simulink library "halin"  (R2021b)
settings: Solver=VariableStepAuto  StartTime=0.0  StopTime=10.0  RelTol=1e-3
undefined symbols (not defined in the file): TRUE
libraries: FVT_lib x37, hcu_lib x31
(part 3 of 4)

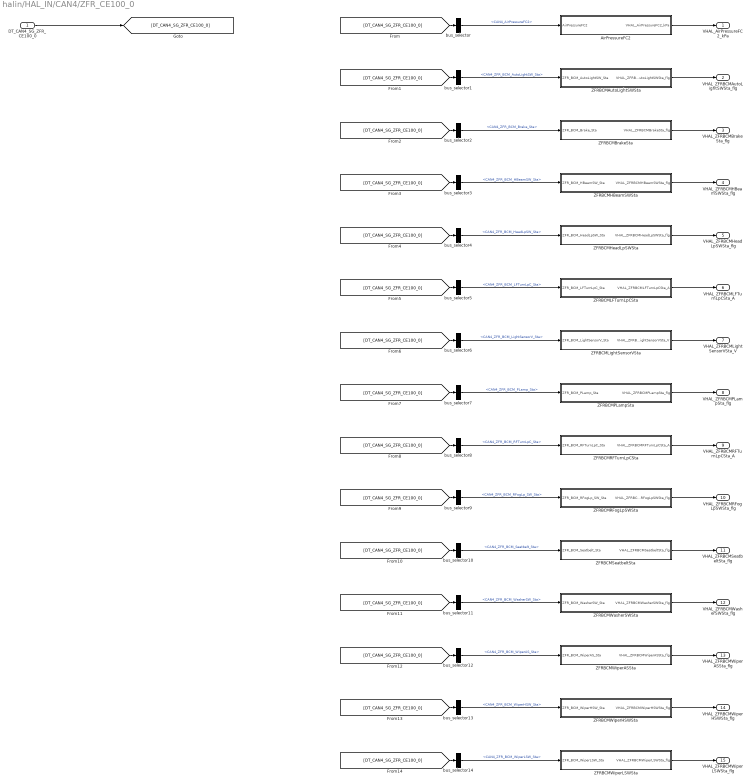
== system halin/HAL_IN/CAN4/ZFR_CE100_0 ==
  DT_CAN4_SG_ZFR_CE100_0 : Inport
  AirPressureFC2 : Subsystem
  ZFRBCMAutoLightSWSta : Subsystem
  ZFRBCMBrakeSta : Subsystem
  ZFRBCMHBeamSWSta : Subsystem
  ZFRBCMHeadLpSWSta : Subsystem
  ZFRBCMLFTurnLpCSta : Subsystem
  ZFRBCMLightSensorVSta : Subsystem
  ZFRBCMPLampSta : Subsystem
  ZFRBCMRFTurnLpCSta : Subsystem
  ZFRBCMRFogLpSWSta : Subsystem
  ZFRBCMSeatbeltSta : Subsystem
  ZFRBCMWasherSWSta : Subsystem
  ZFRBCMWiperASSta : Subsystem
  ZFRBCMWiperHSWSta : Subsystem
  ZFRBCMWiperLSWSta : Subsystem
  bus_selector : BusSelector  OutputSignals=CAN4_AirPressureFC2
  bus_selector1 : BusSelector  OutputSignals=CAN4_ZFR_BCM_AutoLightSW_Sta
  bus_selector10 : BusSelector  OutputSignals=CAN4_ZFR_BCM_Seatbelt_Sta
  bus_selector11 : BusSelector  OutputSignals=CAN4_ZFR_BCM_WasherSW_Sta
  bus_selector12 : BusSelector  OutputSignals=CAN4_ZFR_BCM_WiperAS_Sta
  bus_selector13 : BusSelector  OutputSignals=CAN4_ZFR_BCM_WiperHSW_Sta
  bus_selector14 : BusSelector  OutputSignals=CAN4_ZFR_BCM_WiperLSW_Sta
  bus_selector2 : BusSelector  OutputSignals=CAN4_ZFR_BCM_Brake_Sta
  bus_selector3 : BusSelector  OutputSignals=CAN4_ZFR_BCM_HBeamSW_Sta
  bus_selector4 : BusSelector  OutputSignals=CAN4_ZFR_BCM_HeadLpSW_Sta
  bus_selector5 : BusSelector  OutputSignals=CAN4_ZFR_BCM_LFTurnLpC_Sta
  bus_selector6 : BusSelector  OutputSignals=CAN4_ZFR_BCM_LightSensorV_Sta
  bus_selector7 : BusSelector  OutputSignals=CAN4_ZFR_BCM_PLamp_Sta
  bus_selector8 : BusSelector  OutputSignals=CAN4_ZFR_BCM_RFTurnLpC_Sta
  bus_selector9 : BusSelector  OutputSignals=CAN4_ZFR_BCM_RFogLp_SW_Sta
  VHAL_AirPressureFC2_kPa : Outport
  VHAL_ZFRBCMAutoLightSWSta_flg : Outport  Port=2
  VHAL_ZFRBCMBrakeSta_flg : Outport  Port=3
  VHAL_ZFRBCMHBeamSWSta_flg : Outport  Port=4
  VHAL_ZFRBCMHeadLpSWSta_flg : Outport  Port=5
  VHAL_ZFRBCMLFTurnLpCSta_A : Outport  Port=6
  VHAL_ZFRBCMLightSensorVSta_V : Outport  Port=7
  VHAL_ZFRBCMPLampSta_flg : Outport  Port=8
  VHAL_ZFRBCMRFTurnLpCSta_A : Outport  Port=9
  VHAL_ZFRBCMRFogLpSWSta_flg : Outport  Port=10
  VHAL_ZFRBCMSeatbeltSta_flg : Outport  Port=11
  VHAL_ZFRBCMWasherSWSta_flg : Outport  Port=12
  VHAL_ZFRBCMWiperASSta_flg : Outport  Port=13
  VHAL_ZFRBCMWiperHSWSta_flg : Outport  Port=14
  VHAL_ZFRBCMWiperLSWSta_flg : Outport  Port=15
  wires:
  DT_CAN4_SG_ZFR_CE100_0/1 -> [DT_CAN4_SG_ZFR_CE100_0]
  [DT_CAN4_SG_ZFR_CE100_0] -> bus_selector/1
  bus_selector/1 -> AirPressureFC2/1(AirPressureFC2)  "<CAN4_AirPressureFC2>"
  AirPressureFC2/1(VHAL_AirPressureFC2_kPa) -> VHAL_AirPressureFC2_kPa/1
  [DT_CAN4_SG_ZFR_CE100_0] -> bus_selector1/1
  bus_selector1/1 -> ZFRBCMAutoLightSWSta/1(ZFR_BCM_AutoLightSW_Sta)  "<CAN4_ZFR_BCM_AutoLightSW_Sta>"
  ZFRBCMAutoLightSWSta/1(VHAL_ZFRBCMAutoLightSWSta_flg) -> VHAL_ZFRBCMAutoLightSWSta_flg/1
  [DT_CAN4_SG_ZFR_CE100_0] -> bus_selector2/1
  bus_selector2/1 -> ZFRBCMBrakeSta/1(ZFR_BCM_Brake_Sta)  "<CAN4_ZFR_BCM_Brake_Sta>"
  ZFRBCMBrakeSta/1(VHAL_ZFRBCMBrakeSta_flg) -> VHAL_ZFRBCMBrakeSta_flg/1
  [DT_CAN4_SG_ZFR_CE100_0] -> bus_selector3/1
  bus_selector3/1 -> ZFRBCMHBeamSWSta/1(ZFR_BCM_HBeamSW_Sta)  "<CAN4_ZFR_BCM_HBeamSW_Sta>"
  ZFRBCMHBeamSWSta/1(VHAL_ZFRBCMHBeamSWSta_flg) -> VHAL_ZFRBCMHBeamSWSta_flg/1
  [DT_CAN4_SG_ZFR_CE100_0] -> bus_selector4/1
  bus_selector4/1 -> ZFRBCMHeadLpSWSta/1(ZFR_BCM_HeadLpSW_Sta)  "<CAN4_ZFR_BCM_HeadLpSW_Sta>"
  ZFRBCMHeadLpSWSta/1(VHAL_ZFRBCMHeadLpSWSta_flg) -> VHAL_ZFRBCMHeadLpSWSta_flg/1
  [DT_CAN4_SG_ZFR_CE100_0] -> bus_selector5/1
  bus_selector5/1 -> ZFRBCMLFTurnLpCSta/1(ZFR_BCM_LFTurnLpC_Sta)  "<CAN4_ZFR_BCM_LFTurnLpC_Sta>"
  ZFRBCMLFTurnLpCSta/1(VHAL_ZFRBCMLFTurnLpCSta_A) -> VHAL_ZFRBCMLFTurnLpCSta_A/1
  [DT_CAN4_SG_ZFR_CE100_0] -> bus_selector6/1
  bus_selector6/1 -> ZFRBCMLightSensorVSta/1(ZFR_BCM_LightSensorV_Sta)  "<CAN4_ZFR_BCM_LightSensorV_Sta>"
  ZFRBCMLightSensorVSta/1(VHAL_ZFRBCMLightSensorVSta_V) -> VHAL_ZFRBCMLightSensorVSta_V/1
  [DT_CAN4_SG_ZFR_CE100_0] -> bus_selector7/1
  bus_selector7/1 -> ZFRBCMPLampSta/1(ZFR_BCM_PLamp_Sta)  "<CAN4_ZFR_BCM_PLamp_Sta>"
  ZFRBCMPLampSta/1(VHAL_ZFRBCMPLampSta_flg) -> VHAL_ZFRBCMPLampSta_flg/1
  [DT_CAN4_SG_ZFR_CE100_0] -> bus_selector8/1
  bus_selector8/1 -> ZFRBCMRFTurnLpCSta/1(ZFR_BCM_RFTurnLpC_Sta)  "<CAN4_ZFR_BCM_RFTurnLpC_Sta>"
  ZFRBCMRFTurnLpCSta/1(VHAL_ZFRBCMRFTurnLpCSta_A) -> VHAL_ZFRBCMRFTurnLpCSta_A/1
  [DT_CAN4_SG_ZFR_CE100_0] -> bus_selector9/1
  bus_selector9/1 -> ZFRBCMRFogLpSWSta/1(ZFR_BCM_RFogLp_SW_Sta)  "<CAN4_ZFR_BCM_RFogLp_SW_Sta>"
  ZFRBCMRFogLpSWSta/1(VHAL_ZFRBCMRFogLpSWSta_flg) -> VHAL_ZFRBCMRFogLpSWSta_flg/1
  [DT_CAN4_SG_ZFR_CE100_0] -> bus_selector10/1
  bus_selector10/1 -> ZFRBCMSeatbeltSta/1(ZFR_BCM_Seatbelt_Sta)  "<CAN4_ZFR_BCM_Seatbelt_Sta>"
  ZFRBCMSeatbeltSta/1(VHAL_ZFRBCMSeatbeltSta_flg) -> VHAL_ZFRBCMSeatbeltSta_flg/1
  [DT_CAN4_SG_ZFR_CE100_0] -> bus_selector11/1
  bus_selector11/1 -> ZFRBCMWasherSWSta/1(ZFR_BCM_WasherSW_Sta)  "<CAN4_ZFR_BCM_WasherSW_Sta>"
  ZFRBCMWasherSWSta/1(VHAL_ZFRBCMWasherSWSta_flg) -> VHAL_ZFRBCMWasherSWSta_flg/1
  [DT_CAN4_SG_ZFR_CE100_0] -> bus_selector12/1
  bus_selector12/1 -> ZFRBCMWiperASSta/1(ZFR_BCM_WiperAS_Sta)  "<CAN4_ZFR_BCM_WiperAS_Sta>"
  ZFRBCMWiperASSta/1(VHAL_ZFRBCMWiperASSta_flg) -> VHAL_ZFRBCMWiperASSta_flg/1
  [DT_CAN4_SG_ZFR_CE100_0] -> bus_selector13/1
  bus_selector13/1 -> ZFRBCMWiperHSWSta/1(ZFR_BCM_WiperHSW_Sta)  "<CAN4_ZFR_BCM_WiperHSW_Sta>"
  ZFRBCMWiperHSWSta/1(VHAL_ZFRBCMWiperHSWSta_flg) -> VHAL_ZFRBCMWiperHSWSta_flg/1
  [DT_CAN4_SG_ZFR_CE100_0] -> bus_selector14/1
  bus_selector14/1 -> ZFRBCMWiperLSWSta/1(ZFR_BCM_WiperLSW_Sta)  "<CAN4_ZFR_BCM_WiperLSW_Sta>"
  ZFRBCMWiperLSWSta/1(VHAL_ZFRBCMWiperLSWSta_flg) -> VHAL_ZFRBCMWiperLSWSta_flg/1

== system halin/HAL_IN/CAN4/ZRR_CE100_0 ==
  DT_CAN4_SG_ZRR_CE100_0 : Inport
  ZRRBCMAllDoorSta : Subsystem
  bus_selector : BusSelector  OutputSignals=CAN4_ZRR_BCM_AllDoor_Sta
  VHAL_ZRRBCMAllDoorSta_enum : Outport
  wires:
  DT_CAN4_SG_ZRR_CE100_0/1 -> [DT_CAN4_SG_ZRR_CE100_0]
  [DT_CAN4_SG_ZRR_CE100_0] -> bus_selector/1
  bus_selector/1 -> ZRRBCMAllDoorSta/1(ZRR_BCM_AllDoor_Sta)  "<CAN4_ZRR_BCM_AllDoor_Sta>"
  ZRRBCMAllDoorSta/1(VHAL_ZRRBCMAllDoorSta_enum) -> VHAL_ZRRBCMAllDoorSta_enum/1

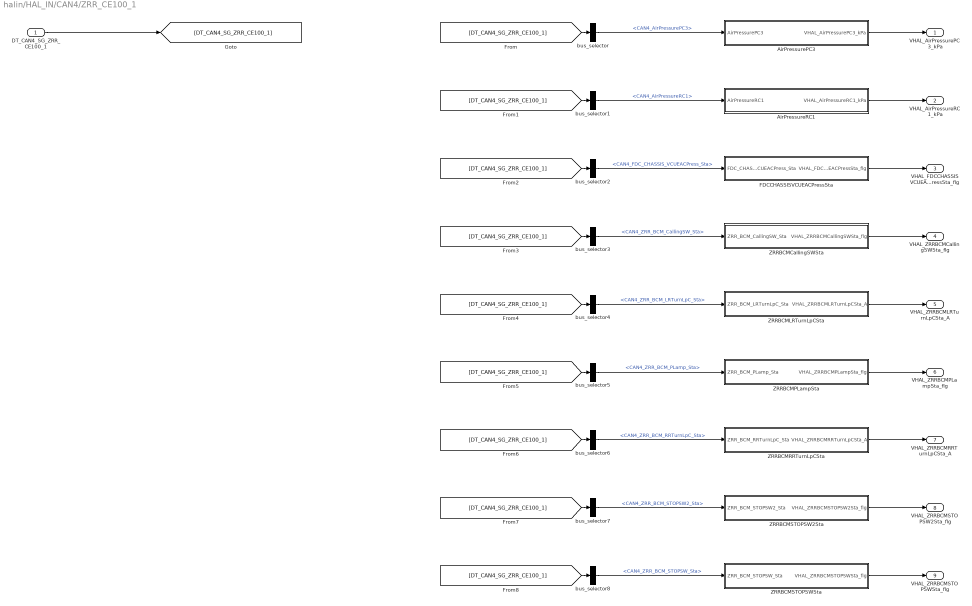
== system halin/HAL_IN/CAN4/ZRR_CE100_1 ==
  DT_CAN4_SG_ZRR_CE100_1 : Inport
  AirPressurePC3 : Subsystem
  AirPressureRC1 : Subsystem
  FDCCHASSISVCUEACPressSta : Subsystem
  ZRRBCMCallingSWSta : Subsystem
  ZRRBCMLRTurnLpCSta : Subsystem
  ZRRBCMPLampSta : Subsystem
  ZRRBCMRRTurnLpCSta : Subsystem
  ZRRBCMSTOPSW2Sta : Subsystem
  ZRRBCMSTOPSWSta : Subsystem
  bus_selector : BusSelector  OutputSignals=CAN4_AirPressurePC3
  bus_selector1 : BusSelector  OutputSignals=CAN4_AirPressureRC1
  bus_selector2 : BusSelector  OutputSignals=CAN4_FDC_CHASSIS_VCUEACPress_Sta
  bus_selector3 : BusSelector  OutputSignals=CAN4_ZRR_BCM_CallingSW_Sta
  bus_selector4 : BusSelector  OutputSignals=CAN4_ZRR_BCM_LRTurnLpC_Sta
  bus_selector5 : BusSelector  OutputSignals=CAN4_ZRR_BCM_PLamp_Sta
  bus_selector6 : BusSelector  OutputSignals=CAN4_ZRR_BCM_RRTurnLpC_Sta
  bus_selector7 : BusSelector  OutputSignals=CAN4_ZRR_BCM_STOPSW2_Sta
  bus_selector8 : BusSelector  OutputSignals=CAN4_ZRR_BCM_STOPSW_Sta
  VHAL_AirPressurePC3_kPa : Outport
  VHAL_AirPressureRC1_kPa : Outport  Port=2
  VHAL_FDCCHASSISVCUEACPressSta_flg : Outport  Port=3
  VHAL_ZRRBCMCallingSWSta_flg : Outport  Port=4
  VHAL_ZRRBCMLRTurnLpCSta_A : Outport  Port=5
  VHAL_ZRRBCMPLampSta_flg : Outport  Port=6
  VHAL_ZRRBCMRRTurnLpCSta_A : Outport  Port=7
  VHAL_ZRRBCMSTOPSW2Sta_flg : Outport  Port=8
  VHAL_ZRRBCMSTOPSWSta_flg : Outport  Port=9
  wires:
  DT_CAN4_SG_ZRR_CE100_1/1 -> [DT_CAN4_SG_ZRR_CE100_1]
  [DT_CAN4_SG_ZRR_CE100_1] -> bus_selector/1
  bus_selector/1 -> AirPressurePC3/1(AirPressurePC3)  "<CAN4_AirPressurePC3>"
  AirPressurePC3/1(VHAL_AirPressurePC3_kPa) -> VHAL_AirPressurePC3_kPa/1
  [DT_CAN4_SG_ZRR_CE100_1] -> bus_selector1/1
  bus_selector1/1 -> AirPressureRC1/1(AirPressureRC1)  "<CAN4_AirPressureRC1>"
  AirPressureRC1/1(VHAL_AirPressureRC1_kPa) -> VHAL_AirPressureRC1_kPa/1
  [DT_CAN4_SG_ZRR_CE100_1] -> bus_selector2/1
  bus_selector2/1 -> FDCCHASSISVCUEACPressSta/1(FDC_CHASSIS_VCUEACPress_Sta)  "<CAN4_FDC_CHASSIS_VCUEACPress_Sta>"
  FDCCHASSISVCUEACPressSta/1(VHAL_FDCCHASSISVCUEACPressSta_flg) -> VHAL_FDCCHASSISVCUEACPressSta_flg/1
  [DT_CAN4_SG_ZRR_CE100_1] -> bus_selector3/1
  bus_selector3/1 -> ZRRBCMCallingSWSta/1(ZRR_BCM_CallingSW_Sta)  "<CAN4_ZRR_BCM_CallingSW_Sta>"
  ZRRBCMCallingSWSta/1(VHAL_ZRRBCMCallingSWSta_flg) -> VHAL_ZRRBCMCallingSWSta_flg/1
  [DT_CAN4_SG_ZRR_CE100_1] -> bus_selector4/1
  bus_selector4/1 -> ZRRBCMLRTurnLpCSta/1(ZRR_BCM_LRTurnLpC_Sta)  "<CAN4_ZRR_BCM_LRTurnLpC_Sta>"
  ZRRBCMLRTurnLpCSta/1(VHAL_ZRRBCMLRTurnLpCSta_A) -> VHAL_ZRRBCMLRTurnLpCSta_A/1
  [DT_CAN4_SG_ZRR_CE100_1] -> bus_selector5/1
  bus_selector5/1 -> ZRRBCMPLampSta/1(ZRR_BCM_PLamp_Sta)  "<CAN4_ZRR_BCM_PLamp_Sta>"
  ZRRBCMPLampSta/1(VHAL_ZRRBCMPLampSta_flg) -> VHAL_ZRRBCMPLampSta_flg/1
  [DT_CAN4_SG_ZRR_CE100_1] -> bus_selector6/1
  bus_selector6/1 -> ZRRBCMRRTurnLpCSta/1(ZRR_BCM_RRTurnLpC_Sta)  "<CAN4_ZRR_BCM_RRTurnLpC_Sta>"
  ZRRBCMRRTurnLpCSta/1(VHAL_ZRRBCMRRTurnLpCSta_A) -> VHAL_ZRRBCMRRTurnLpCSta_A/1
  [DT_CAN4_SG_ZRR_CE100_1] -> bus_selector7/1
  bus_selector7/1 -> ZRRBCMSTOPSW2Sta/1(ZRR_BCM_STOPSW2_Sta)  "<CAN4_ZRR_BCM_STOPSW2_Sta>"
  ZRRBCMSTOPSW2Sta/1(VHAL_ZRRBCMSTOPSW2Sta_flg) -> VHAL_ZRRBCMSTOPSW2Sta_flg/1
  [DT_CAN4_SG_ZRR_CE100_1] -> bus_selector8/1
  bus_selector8/1 -> ZRRBCMSTOPSWSta/1(ZRR_BCM_STOPSW_Sta)  "<CAN4_ZRR_BCM_STOPSW_Sta>"
  ZRRBCMSTOPSWSta/1(VHAL_ZRRBCMSTOPSWSta_flg) -> VHAL_ZRRBCMSTOPSWSta_flg/1

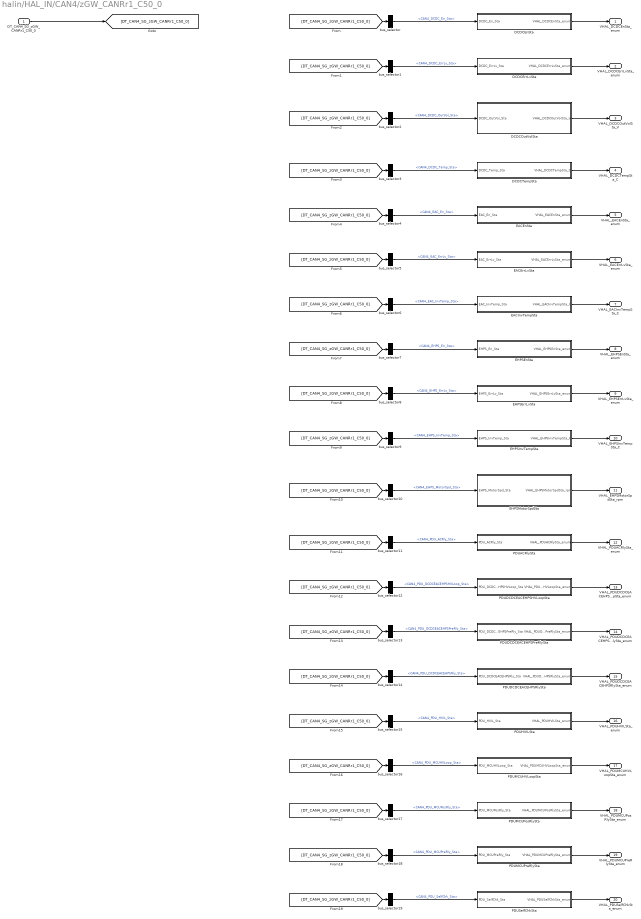
== system halin/HAL_IN/CAN4/zGW_CANRr1_C50_0 ==
  DT_CAN4_SG_zGW_CANRr1_C50_0 : Inport
  DCDCEnSta : Subsystem
  DCDCErrLvSta : Subsystem
  DCDCOutVolSta : Subsystem
  DCDCTempSta : Subsystem
  EACEnSta : Subsystem
  EACErrLvSta : Subsystem
  EACInvTempSta : Subsystem
  EHPSEnSta : Subsystem
  EHPSErrLvSta : Subsystem
  EHPSInvTempSta : Subsystem
  EHPSMotorSpdSta : Subsystem
  PDUACRlySta : Subsystem
  PDUDCDCEACEHPSHVLoopSta : Subsystem
  PDUDCDCEACEHPSPreRlySta : Subsystem
  PDUDCDCEACEHPSRlySta : Subsystem
  PDUHVILSta : Subsystem
  PDUMCUHVLoopSta : Subsystem
  PDUMCUPosRlySta : Subsystem
  PDUMCUPreRlySta : Subsystem
  PDUSelfChkSta : Subsystem
  bus_selector : BusSelector  OutputSignals=CAN4_DCDC_En_Sta
  bus_selector1 : BusSelector  OutputSignals=CAN4_DCDC_ErrLv_Sta
  bus_selector10 : BusSelector  OutputSignals=CAN4_EHPS_MotorSpd_Sta
  bus_selector11 : BusSelector  OutputSignals=CAN4_PDU_ACRly_Sta
  bus_selector12 : BusSelector  OutputSignals=CAN4_PDU_DCDCEACEHPSHVLoop_Sta
  bus_selector13 : BusSelector  OutputSignals=CAN4_PDU_DCDCEACEHPSPreRly_Sta
  bus_selector14 : BusSelector  OutputSignals=CAN4_PDU_DCDCEACEHPSRly_Sta
  bus_selector15 : BusSelector  OutputSignals=CAN4_PDU_HVIL_Sta
  bus_selector16 : BusSelector  OutputSignals=CAN4_PDU_MCUHVLoop_Sta
  bus_selector17 : BusSelector  OutputSignals=CAN4_PDU_MCUPosRly_Sta
  bus_selector18 : BusSelector  OutputSignals=CAN4_PDU_MCUPreRly_Sta
  bus_selector19 : BusSelector  OutputSignals=CAN4_PDU_SelfChk_Sta
  bus_selector2 : BusSelector  OutputSignals=CAN4_DCDC_OutVol_Sta
  bus_selector3 : BusSelector  OutputSignals=CAN4_DCDC_Temp_Sta
  bus_selector4 : BusSelector  OutputSignals=CAN4_EAC_En_Sta
  bus_selector5 : BusSelector  OutputSignals=CAN4_EAC_ErrLv_Sta
  bus_selector6 : BusSelector  OutputSignals=CAN4_EAC_InvTemp_Sta
  bus_selector7 : BusSelector  OutputSignals=CAN4_EHPS_En_Sta
  bus_selector8 : BusSelector  OutputSignals=CAN4_EHPS_ErrLv_Sta
  bus_selector9 : BusSelector  OutputSignals=CAN4_EHPS_InvTemp_Sta
  VHAL_DCDCEnSta_enum : Outport
  VHAL_DCDCErrLvSta_enum : Outport  Port=2
  VHAL_DCDCOutVolSta_V : Outport  Port=3
  VHAL_DCDCTempSta_C : Outport  Port=4
  VHAL_EACEnSta_enum : Outport  Port=5
  VHAL_EACErrLvSta_enum : Outport  Port=6
  VHAL_EACInvTempSta_C : Outport  Port=7
  VHAL_EHPSEnSta_enum : Outport  Port=8
  VHAL_EHPSErrLvSta_enum : Outport  Port=9
  VHAL_EHPSInvTempSta_C : Outport  Port=10
  VHAL_EHPSMotorSpdSta_rpm : Outport  Port=11
  VHAL_PDUACRlySta_enum : Outport  Port=12
  VHAL_PDUDCDCEACEHPSHVLoopSta_enum : Outport  Port=13
  VHAL_PDUDCDCEACEHPSPreRlySta_enum : Outport  Port=14
  VHAL_PDUDCDCEACEHPSRlySta_enum : Outport  Port=15
  VHAL_PDUHVILSta_enum : Outport  Port=16
  VHAL_PDUMCUHVLoopSta_enum : Outport  Port=17
  VHAL_PDUMCUPosRlySta_enum : Outport  Port=18
  VHAL_PDUMCUPreRlySta_enum : Outport  Port=19
  VHAL_PDUSelfChkSta_enum : Outport  Port=20
  wires:
  DT_CAN4_SG_zGW_CANRr1_C50_0/1 -> [DT_CAN4_SG_zGW_CANRr1_C50_0]
  [DT_CAN4_SG_zGW_CANRr1_C50_0] -> bus_selector/1
  bus_selector/1 -> DCDCEnSta/1(DCDC_En_Sta)  "<CAN4_DCDC_En_Sta>"
  DCDCEnSta/1(VHAL_DCDCEnSta_enum) -> VHAL_DCDCEnSta_enum/1
  [DT_CAN4_SG_zGW_CANRr1_C50_0] -> bus_selector1/1
  bus_selector1/1 -> DCDCErrLvSta/1(DCDC_ErrLv_Sta)  "<CAN4_DCDC_ErrLv_Sta>"
  DCDCErrLvSta/1(VHAL_DCDCErrLvSta_enum) -> VHAL_DCDCErrLvSta_enum/1
  [DT_CAN4_SG_zGW_CANRr1_C50_0] -> bus_selector2/1
  bus_selector2/1 -> DCDCOutVolSta/1(DCDC_OutVol_Sta)  "<CAN4_DCDC_OutVol_Sta>"
  DCDCOutVolSta/1(VHAL_DCDCOutVolSta_V) -> VHAL_DCDCOutVolSta_V/1
  [DT_CAN4_SG_zGW_CANRr1_C50_0] -> bus_selector3/1
  bus_selector3/1 -> DCDCTempSta/1(DCDC_Temp_Sta)  "<CAN4_DCDC_Temp_Sta>"
  DCDCTempSta/1(VHAL_DCDCTempSta_C) -> VHAL_DCDCTempSta_C/1
  [DT_CAN4_SG_zGW_CANRr1_C50_0] -> bus_selector4/1
  bus_selector4/1 -> EACEnSta/1(EAC_En_Sta)  "<CAN4_EAC_En_Sta>"
  EACEnSta/1(VHAL_EACEnSta_enum) -> VHAL_EACEnSta_enum/1
  [DT_CAN4_SG_zGW_CANRr1_C50_0] -> bus_selector5/1
  bus_selector5/1 -> EACErrLvSta/1(EAC_ErrLv_Sta)  "<CAN4_EAC_ErrLv_Sta>"
  EACErrLvSta/1(VHAL_EACErrLvSta_enum) -> VHAL_EACErrLvSta_enum/1
  [DT_CAN4_SG_zGW_CANRr1_C50_0] -> bus_selector6/1
  bus_selector6/1 -> EACInvTempSta/1(EAC_InvTemp_Sta)  "<CAN4_EAC_InvTemp_Sta>"
  EACInvTempSta/1(VHAL_EACInvTempSta_C) -> VHAL_EACInvTempSta_C/1
  [DT_CAN4_SG_zGW_CANRr1_C50_0] -> bus_selector7/1
  bus_selector7/1 -> EHPSEnSta/1(EHPS_En_Sta)  "<CAN4_EHPS_En_Sta>"
  EHPSEnSta/1(VHAL_EHPSEnSta_enum) -> VHAL_EHPSEnSta_enum/1
  [DT_CAN4_SG_zGW_CANRr1_C50_0] -> bus_selector8/1
  bus_selector8/1 -> EHPSErrLvSta/1(EHPS_ErrLv_Sta)  "<CAN4_EHPS_ErrLv_Sta>"
  EHPSErrLvSta/1(VHAL_EHPSErrLvSta_enum) -> VHAL_EHPSErrLvSta_enum/1
  [DT_CAN4_SG_zGW_CANRr1_C50_0] -> bus_selector9/1
  bus_selector9/1 -> EHPSInvTempSta/1(EHPS_InvTemp_Sta)  "<CAN4_EHPS_InvTemp_Sta>"
  EHPSInvTempSta/1(VHAL_EHPSInvTempSta_C) -> VHAL_EHPSInvTempSta_C/1
  [DT_CAN4_SG_zGW_CANRr1_C50_0] -> bus_selector10/1
  bus_selector10/1 -> EHPSMotorSpdSta/1(EHPS_MotorSpd_Sta)  "<CAN4_EHPS_MotorSpd_Sta>"
  EHPSMotorSpdSta/1(VHAL_EHPSMotorSpdSta_rpm) -> VHAL_EHPSMotorSpdSta_rpm/1
  [DT_CAN4_SG_zGW_CANRr1_C50_0] -> bus_selector11/1
  bus_selector11/1 -> PDUACRlySta/1(PDU_ACRly_Sta)  "<CAN4_PDU_ACRly_Sta>"
  PDUACRlySta/1(VHAL_PDUACRlySta_enum) -> VHAL_PDUACRlySta_enum/1
  [DT_CAN4_SG_zGW_CANRr1_C50_0] -> bus_selector12/1
  bus_selector12/1 -> PDUDCDCEACEHPSHVLoopSta/1(PDU_DCDCEACEHPSHVLoop_Sta)  "<CAN4_PDU_DCDCEACEHPSHVLoop_Sta>"
  PDUDCDCEACEHPSHVLoopSta/1(VHAL_PDUDCDCEACEHPSHVLoopSta_enum) -> VHAL_PDUDCDCEACEHPSHVLoopSta_enum/1
  [DT_CAN4_SG_zGW_CANRr1_C50_0] -> bus_selector13/1
  bus_selector13/1 -> PDUDCDCEACEHPSPreRlySta/1(PDU_DCDCEACEHPSPreRly_Sta)  "<CAN4_PDU_DCDCEACEHPSPreRly_Sta>"
  PDUDCDCEACEHPSPreRlySta/1(VHAL_PDUDCDCEACEHPSPreRlySta_enum) -> VHAL_PDUDCDCEACEHPSPreRlySta_enum/1
  [DT_CAN4_SG_zGW_CANRr1_C50_0] -> bus_selector14/1
  bus_selector14/1 -> PDUDCDCEACEHPSRlySta/1(PDU_DCDCEACEHPSRly_Sta)  "<CAN4_PDU_DCDCEACEHPSRly_Sta>"
  PDUDCDCEACEHPSRlySta/1(VHAL_PDUDCDCEACEHPSRlySta_enum) -> VHAL_PDUDCDCEACEHPSRlySta_enum/1
  [DT_CAN4_SG_zGW_CANRr1_C50_0] -> bus_selector15/1
  bus_selector15/1 -> PDUHVILSta/1(PDU_HVIL_Sta)  "<CAN4_PDU_HVIL_Sta>"
  PDUHVILSta/1(VHAL_PDUHVILSta_enum) -> VHAL_PDUHVILSta_enum/1
  [DT_CAN4_SG_zGW_CANRr1_C50_0] -> bus_selector16/1
  bus_selector16/1 -> PDUMCUHVLoopSta/1(PDU_MCUHVLoop_Sta)  "<CAN4_PDU_MCUHVLoop_Sta>"
  PDUMCUHVLoopSta/1(VHAL_PDUMCUHVLoopSta_enum) -> VHAL_PDUMCUHVLoopSta_enum/1
  [DT_CAN4_SG_zGW_CANRr1_C50_0] -> bus_selector17/1
  bus_selector17/1 -> PDUMCUPosRlySta/1(PDU_MCUPosRly_Sta)  "<CAN4_PDU_MCUPosRly_Sta>"
  PDUMCUPosRlySta/1(VHAL_PDUMCUPosRlySta_enum) -> VHAL_PDUMCUPosRlySta_enum/1
  [DT_CAN4_SG_zGW_CANRr1_C50_0] -> bus_selector18/1
  bus_selector18/1 -> PDUMCUPreRlySta/1(PDU_MCUPreRly_Sta)  "<CAN4_PDU_MCUPreRly_Sta>"
  PDUMCUPreRlySta/1(VHAL_PDUMCUPreRlySta_enum) -> VHAL_PDUMCUPreRlySta_enum/1
  [DT_CAN4_SG_zGW_CANRr1_C50_0] -> bus_selector19/1
  bus_selector19/1 -> PDUSelfChkSta/1(PDU_SelfChk_Sta)  "<CAN4_PDU_SelfChk_Sta>"
  PDUSelfChkSta/1(VHAL_PDUSelfChkSta_enum) -> VHAL_PDUSelfChkSta_enum/1

== system halin/HAL_IN/CAN1/AC_BTMS_C1000_0/ACAmbTemp ==
  ACAmbTemp : Inport
  UnitConverter : DataTypeConversion  OutDataTypeStr=uint16
  convert_in : FVT_lib/hal/convert_in  gain=0.1  offset=-20
  VHAL_ACAmbTemp_C : Outport
  wires:
  convert_in/1 -> VHAL_ACAmbTemp_C/1
  UnitConverter/1 -> convert_in/1
  ACAmbTemp/1 -> UnitConverter/1

== system halin/HAL_IN/CAN1/AC_BTMS_C1000_1/ACFanSpdSta ==
  ACFanSpdSta : Inport
  UnitConverter : DataTypeConversion  OutDataTypeStr=uint8
  VHAL_ACFanSpdSta_enum : Outport
  wires:
  UnitConverter/1 -> VHAL_ACFanSpdSta_enum/1
  ACFanSpdSta/1 -> UnitConverter/1

== system halin/HAL_IN/CAN1/AC_BTMS_C1000_4/TM2BFaultCode ==
  TM2BFaultCode : Inport
  UnitConverter : DataTypeConversion  OutDataTypeStr=uint8
  VHAL_TM2BFaultCode_enum : Outport
  wires:
  UnitConverter/1 -> VHAL_TM2BFaultCode_enum/1
  TM2BFaultCode/1 -> UnitConverter/1

== system halin/HAL_IN/CAN1/AC_BTMS_C5000_0/ACTempSetSta ==
  ACTempSetSta : Inport
  UnitConverter : DataTypeConversion  OutDataTypeStr=uint8
  convert_in : FVT_lib/hal/convert_in  gain=1  offset=-40
  VHAL_ACTempSetSta_C : Outport
  wires:
  convert_in/1 -> VHAL_ACTempSetSta_C/1
  UnitConverter/1 -> convert_in/1
  ACTempSetSta/1 -> UnitConverter/1

== system halin/HAL_IN/CAN1/ASC1_A/ASC1KneelingInfo ==
  ASC1KneelingInfo : Inport
  UnitConverter : DataTypeConversion  OutDataTypeStr=uint8
  VHAL_ASC1KneelingInfo_enum : Outport
  wires:
  UnitConverter/1 -> VHAL_ASC1KneelingInfo_enum/1
  ASC1KneelingInfo/1 -> UnitConverter/1

== system halin/HAL_IN/CAN1/EBC1/ABSFullyOper ==
  ABSFullyOper : Inport
  UnitConverter : DataTypeConversion  OutDataTypeStr=uint8
  VHAL_ABSFullyOper_enum : Outport
  wires:
  UnitConverter/1 -> VHAL_ABSFullyOper_enum/1
  ABSFullyOper/1 -> UnitConverter/1

== system halin/HAL_IN/CAN1/EBC1/ABSOffroadSw ==
  ABSOffroadSw : Inport
  UnitConverter : DataTypeConversion  OutDataTypeStr=uint8
  VHAL_ABSOffroadSw_enum : Outport
  wires:
  UnitConverter/1 -> VHAL_ABSOffroadSw_enum/1
  ABSOffroadSw/1 -> UnitConverter/1

== system halin/HAL_IN/CAN1/EBC1/ASRBrakeCtrlAtc ==
  ASRBrakeCtrlAtc : Inport
  UnitConverter : DataTypeConversion  OutDataTypeStr=uint8
  VHAL_ASRBrakeCtrlAtc_enum : Outport
  wires:
  UnitConverter/1 -> VHAL_ASRBrakeCtrlAtc_enum/1
  ASRBrakeCtrlAtc/1 -> UnitConverter/1

== system halin/HAL_IN/CAN1/EBC1/ASREngCtrlAtc ==
  ASREngCtrlAtc : Inport
  UnitConverter : DataTypeConversion  OutDataTypeStr=uint8
  VHAL_ASREngCtrlAtc_enum : Outport
  wires:
  UnitConverter/1 -> VHAL_ASREngCtrlAtc_enum/1
  ASREngCtrlAtc/1 -> UnitConverter/1

== system halin/HAL_IN/CAN1/EBC1/ASRHillHolderSw ==
  ASRHillHolderSw : Inport
  UnitConverter : DataTypeConversion  OutDataTypeStr=uint8
  VHAL_ASRHillHolderSw_enum : Outport
  wires:
  UnitConverter/1 -> VHAL_ASRHillHolderSw_enum/1
  ASRHillHolderSw/1 -> UnitConverter/1

== system halin/HAL_IN/CAN1/EBC1/ASROffroadSw ==
  ASROffroadSw : Inport
  UnitConverter : DataTypeConversion  OutDataTypeStr=uint8
  VHAL_ASROffroadSw_enum : Outport
  wires:
  UnitConverter/1 -> VHAL_ASROffroadSw_enum/1
  ASROffroadSw/1 -> UnitConverter/1

== system halin/HAL_IN/CAN1/EBC1/ATCASRInfoSig ==
  ATCASRInfoSig : Inport
  UnitConverter : DataTypeConversion  OutDataTypeStr=uint8
  VHAL_ATCASRInfoSig_enum : Outport
  wires:
  UnitConverter/1 -> VHAL_ATCASRInfoSig_enum/1
  ATCASRInfoSig/1 -> UnitConverter/1

== system halin/HAL_IN/CAN1/EBC1/AcltrInterlockSw ==
  AcltrInterlockSw : Inport
  UnitConverter : DataTypeConversion  OutDataTypeStr=uint8
  VHAL_AcltrInterlockSw_enum : Outport
  wires:
  UnitConverter/1 -> VHAL_AcltrInterlockSw_enum/1
  AcltrInterlockSw/1 -> UnitConverter/1

== system halin/HAL_IN/CAN1/EBC1/AntiLBrakABSAct ==
  AntiLBrakABSAct : Inport
  UnitConverter : DataTypeConversion  OutDataTypeStr=uint8
  VHAL_AntiLBrakABSAct_enum : Outport
  wires:
  UnitConverter/1 -> VHAL_AntiLBrakABSAct_enum/1
  AntiLBrakABSAct/1 -> UnitConverter/1

== system halin/HAL_IN/CAN1/EBC1/BrakePedalPos ==
  BrakePedalPos : Inport
  UnitConverter : DataTypeConversion  OutDataTypeStr=uint8
  convert_in : FVT_lib/hal/convert_in  gain=0.4  offset=0
  VHAL_BrakePedalPos_pct : Outport
  wires:
  convert_in/1 -> VHAL_BrakePedalPos_pct/1
  UnitConverter/1 -> convert_in/1
  BrakePedalPos/1 -> UnitConverter/1

== system halin/HAL_IN/CAN1/EBC1/EBSAmWarnLampSta ==
  EBSAmWarnLampSta : Inport
  UnitConverter : DataTypeConversion  OutDataTypeStr=uint8
  VHAL_EBSAmWarnLampSta_enum : Outport
  wires:
  UnitConverter/1 -> VHAL_EBSAmWarnLampSta_enum/1
  EBSAmWarnLampSta/1 -> UnitConverter/1

== system halin/HAL_IN/CAN1/EBC1/EBSBrakeSw ==
  EBSBrakeSw : Inport
  UnitConverter : DataTypeConversion  OutDataTypeStr=uint8
  VHAL_EBSBrakeSw_enum : Outport
  wires:
  UnitConverter/1 -> VHAL_EBSBrakeSw_enum/1
  EBSBrakeSw/1 -> UnitConverter/1

== system halin/HAL_IN/CAN1/EBC1/EBSRedWarnLampSta ==
  EBSRedWarnLampSta : Inport
  UnitConverter : DataTypeConversion  OutDataTypeStr=uint8
  VHAL_EBSRedWarnLampSta_enum : Outport
  wires:
  UnitConverter/1 -> VHAL_EBSRedWarnLampSta_enum/1
  EBSRedWarnLampSta/1 -> UnitConverter/1

== system halin/HAL_IN/CAN1/EBC1/EngAuxShutdownSw ==
  EngAuxShutdownSw : Inport
  UnitConverter : DataTypeConversion  OutDataTypeStr=uint8
  VHAL_EngAuxShutdownSw_enum : Outport
  wires:
  UnitConverter/1 -> VHAL_EngAuxShutdownSw_enum/1
  EngAuxShutdownSw/1 -> UnitConverter/1

== system halin/HAL_IN/CAN1/EBC1/EngDerateSw ==
  EngDerateSw : Inport
  UnitConverter : DataTypeConversion  OutDataTypeStr=uint8
  VHAL_EngDerateSw_enum : Outport
  wires:
  UnitConverter/1 -> VHAL_EngDerateSw_enum/1
  EngDerateSw/1 -> UnitConverter/1

== system halin/HAL_IN/CAN1/EBC1/EngRetSel ==
  EngRetSel : Inport
  UnitConverter : DataTypeConversion  OutDataTypeStr=uint8
  convert_in : FVT_lib/hal/convert_in  gain=0.4  offset=0
  VHAL_EngRetSel_pct : Outport
  wires:
  convert_in/1 -> VHAL_EngRetSel_pct/1
  UnitConverter/1 -> convert_in/1
  EngRetSel/1 -> UnitConverter/1

== system halin/HAL_IN/CAN1/EBC1/HaltBrakeSw ==
  HaltBrakeSw : Inport
  UnitConverter : DataTypeConversion  OutDataTypeStr=uint8
  VHAL_HaltBrakeSw_enum : Outport
  wires:
  UnitConverter/1 -> VHAL_HaltBrakeSw_enum/1
  HaltBrakeSw/1 -> UnitConverter/1

== system halin/HAL_IN/CAN1/EBC1/RmAccelEnSw ==
  RmAccelEnSw : Inport
  UnitConverter : DataTypeConversion  OutDataTypeStr=uint8
  VHAL_RmAccelEnSw_enum : Outport
  wires:
  UnitConverter/1 -> VHAL_RmAccelEnSw_enum/1
  RmAccelEnSw/1 -> UnitConverter/1

== system halin/HAL_IN/CAN1/EBC1/SACtrlBrakeCtrl ==
  SACtrlBrakeCtrl : Inport
  UnitConverter : DataTypeConversion  OutDataTypeStr=uint8
  VHAL_SACtrlBrakeCtrl_SA : Outport
  wires:
  UnitConverter/1 -> VHAL_SACtrlBrakeCtrl_SA/1
  SACtrlBrakeCtrl/1 -> UnitConverter/1

== system halin/HAL_IN/CAN1/EBC1/TractCtrlOvrSw ==
  TractCtrlOvrSw : Inport
  UnitConverter : DataTypeConversion  OutDataTypeStr=uint8
  VHAL_TractCtrlOvrSw_enum : Outport
  wires:
  UnitConverter/1 -> VHAL_TractCtrlOvrSw_enum/1
  TractCtrlOvrSw/1 -> UnitConverter/1

== system halin/HAL_IN/CAN1/EBC1/TrailerABSSta ==
  TrailerABSSta : Inport
  UnitConverter : DataTypeConversion  OutDataTypeStr=uint8
  VHAL_TrailerABSSta_enum : Outport
  wires:
  UnitConverter/1 -> VHAL_TrailerABSSta_enum/1
  TrailerABSSta/1 -> UnitConverter/1

== system halin/HAL_IN/CAN1/EBC1/TrailerABSWarnSig ==
  TrailerABSWarnSig : Inport
  UnitConverter : DataTypeConversion  OutDataTypeStr=uint8
  VHAL_TrailerABSWarnSig_enum : Outport
  wires:
  UnitConverter/1 -> VHAL_TrailerABSWarnSig_enum/1
  TrailerABSWarnSig/1 -> UnitConverter/1

== system halin/HAL_IN/CAN1/EBC2/FASpeed ==
  FASpeed : Inport
  UnitConverter : DataTypeConversion  OutDataTypeStr=uint16
  convert_in : FVT_lib/hal/convert_in  gain=0.0039062  offset=0
  VHAL_FASpeed_kph : Outport
  wires:
  convert_in/1 -> VHAL_FASpeed_kph/1
  UnitConverter/1 -> convert_in/1
  FASpeed/1 -> UnitConverter/1

== system halin/HAL_IN/CAN1/EBC2/RelaSpdFALWheel ==
  RelaSpdFALWheel : Inport
  UnitConverter : DataTypeConversion  OutDataTypeStr=uint8
  convert_in : FVT_lib/hal/convert_in  gain=0.0625  offset=-7.8125
  VHAL_RelaSpdFALWheel_kph : Outport
  wires:
  convert_in/1 -> VHAL_RelaSpdFALWheel_kph/1
  UnitConverter/1 -> convert_in/1
  RelaSpdFALWheel/1 -> UnitConverter/1

== system halin/HAL_IN/CAN1/EBC2/RelaSpdFARWheel ==
  RelaSpdFARWheel : Inport
  UnitConverter : DataTypeConversion  OutDataTypeStr=uint8
  convert_in : FVT_lib/hal/convert_in  gain=0.0625  offset=-7.8125
  VHAL_RelaSpdFARWheel_kph : Outport
  wires:
  convert_in/1 -> VHAL_RelaSpdFARWheel_kph/1
  UnitConverter/1 -> convert_in/1
  RelaSpdFARWheel/1 -> UnitConverter/1

== system halin/HAL_IN/CAN1/EBC5/BrkTempeWarn ==
  BrkTempeWarn : Inport
  UnitConverter : DataTypeConversion  OutDataTypeStr=uint8
  VHAL_BrkTempeWarn_enum : Outport
  wires:
  UnitConverter/1 -> VHAL_BrkTempeWarn_enum/1
  BrkTempeWarn/1 -> UnitConverter/1

== system halin/HAL_IN/CAN1/EBC5/FndBrkUse ==
  FndBrkUse : Inport
  UnitConverter : DataTypeConversion  OutDataTypeStr=uint8
  VHAL_FndBrkUse_enum : Outport
  wires:
  UnitConverter/1 -> VHAL_FndBrkUse_enum/1
  FndBrkUse/1 -> UnitConverter/1

== system halin/HAL_IN/CAN1/EBC5/HaltBrkMode ==
  HaltBrkMode : Inport
  UnitConverter : DataTypeConversion  OutDataTypeStr=uint8
  VHAL_HaltBrkMode_enum : Outport
  wires:
  UnitConverter/1 -> VHAL_HaltBrkMode_enum/1
  HaltBrkMode/1 -> UnitConverter/1

== system halin/HAL_IN/CAN1/EBC5/HillHolderMode ==
  HillHolderMode : Inport
  UnitConverter : DataTypeConversion  OutDataTypeStr=uint8
  VHAL_HillHolderMode_enum : Outport
  wires:
  UnitConverter/1 -> VHAL_HillHolderMode_enum/1
  HillHolderMode/1 -> UnitConverter/1

== system halin/HAL_IN/CAN1/EBC5/ParkBrkActuFAct ==
  ParkBrkActuFAct : Inport
  UnitConverter : DataTypeConversion  OutDataTypeStr=uint8
  VHAL_ParkBrkActuFAct_enum : Outport
  wires:
  UnitConverter/1 -> VHAL_ParkBrkActuFAct_enum/1
  ParkBrkActuFAct/1 -> UnitConverter/1

== system halin/HAL_IN/CAN1/EBC5/XBRAcltnLimit ==
  XBRAcltnLimit : Inport
  UnitConverter : DataTypeConversion  OutDataTypeStr=uint8
  convert_in : FVT_lib/hal/convert_in  gain=0.1  offset=-12.5
  VHAL_XBRAcltnLimit_mps2 : Outport
  wires:
  convert_in/1 -> VHAL_XBRAcltnLimit_mps2/1
  UnitConverter/1 -> convert_in/1
  XBRAcltnLimit/1 -> UnitConverter/1

== system halin/HAL_IN/CAN1/EBC5/XBRActtrlMode ==
  XBRActtrlMode : Inport
  UnitConverter : DataTypeConversion  OutDataTypeStr=uint8
  VHAL_XBRActtrlMode_enum : Outport
  wires:
  UnitConverter/1 -> VHAL_XBRActtrlMode_enum/1
  XBRActtrlMode/1 -> UnitConverter/1

== system halin/HAL_IN/CAN1/EBC5/XBRSysSta ==
  XBRSysSta : Inport
  UnitConverter : DataTypeConversion  OutDataTypeStr=uint8
  VHAL_XBRSysSta_enum : Outport
  wires:
  UnitConverter/1 -> VHAL_XBRSysSta_enum/1
  XBRSysSta/1 -> UnitConverter/1

== system halin/HAL_IN/CAN1/ECAS_DM1/ECASAWarmLampSta ==
  ECASAWarmLampSta : Inport
  UnitConverter : DataTypeConversion  OutDataTypeStr=uint8
  VHAL_ECASAWarmLampSta_enum : Outport
  wires:
  UnitConverter/1 -> VHAL_ECASAWarmLampSta_enum/1
  ECASAWarmLampSta/1 -> UnitConverter/1

== system halin/HAL_IN/CAN1/EMC1_EM1/EM1CS ==
  EM1CS : Inport
  UnitConverter : DataTypeConversion  OutDataTypeStr=uint8
  VHAL_EM1CS_enum : Outport
  wires:
  UnitConverter/1 -> VHAL_EM1CS_enum/1
  EM1CS/1 -> UnitConverter/1

== system halin/HAL_IN/CAN1/EMC1_EM1/EM1Cnt ==
  EM1Cnt : Inport
  UnitConverter : DataTypeConversion  OutDataTypeStr=uint8
  VHAL_EM1Cnt_enum : Outport
  wires:
  UnitConverter/1 -> VHAL_EM1Cnt_enum/1
  EM1Cnt/1 -> UnitConverter/1

== system halin/HAL_IN/CAN1/EMC1_EM1/EM1OvrCtrlMBrk ==
  EM1OvrCtrlMBrk : Inport
  UnitConverter : DataTypeConversion  OutDataTypeStr=uint8
  VHAL_EM1OvrCtrlMBrk_enum : Outport
  wires:
  UnitConverter/1 -> VHAL_EM1OvrCtrlMBrk_enum/1
  EM1OvrCtrlMBrk/1 -> UnitConverter/1

== system halin/HAL_IN/CAN1/EMC1_EM1/EM1OvrCtrlMDriv ==
  EM1OvrCtrlMDriv : Inport
  UnitConverter : DataTypeConversion  OutDataTypeStr=uint8
  VHAL_EM1OvrCtrlMDriv_enum : Outport
  wires:
  UnitConverter/1 -> VHAL_EM1OvrCtrlMDriv_enum/1
  EM1OvrCtrlMDriv/1 -> UnitConverter/1

== system halin/HAL_IN/CAN1/EMC1_EM1/EM1OvrCtrlMPriBrk ==
  EM1OvrCtrlMPriBrk : Inport
  UnitConverter : DataTypeConversion  OutDataTypeStr=uint8
  VHAL_EM1OvrCtrlMPriBrk_enum : Outport
  wires:
  UnitConverter/1 -> VHAL_EM1OvrCtrlMPriBrk_enum/1
  EM1OvrCtrlMPriBrk/1 -> UnitConverter/1

== system halin/HAL_IN/CAN1/EMC1_EM1/EM1ReqTorqHRlsBrk ==
  EM1ReqTorqHRlsBrk : Inport
  UnitConverter : DataTypeConversion  OutDataTypeStr=uint8
  VHAL_EM1ReqTorqHRlsBrk_pct : Outport
  wires:
  UnitConverter/1 -> VHAL_EM1ReqTorqHRlsBrk_pct/1
  EM1ReqTorqHRlsBrk/1 -> UnitConverter/1

== system halin/HAL_IN/CAN1/EMC1_EM1/EM1ReqTorqHRlsDri ==
  EM1ReqTorqHRlsDri : Inport
  UnitConverter : DataTypeConversion  OutDataTypeStr=uint8
  VHAL_EM1ReqTorqHRlsDri_pct : Outport
  wires:
  UnitConverter/1 -> VHAL_EM1ReqTorqHRlsDri_pct/1
  EM1ReqTorqHRlsDri/1 -> UnitConverter/1

== system halin/HAL_IN/CAN1/EMC1_EM1/EM1ReqTorqLimBrk ==
  EM1ReqTorqLimBrk : Inport
  UnitConverter : DataTypeConversion  OutDataTypeStr=uint8
  convert_in : FVT_lib/hal/convert_in  gain=1  offset=-125
  VHAL_EM1ReqTorqLimBrk_pct : Outport
  wires:
  convert_in/1 -> VHAL_EM1ReqTorqLimBrk_pct/1
  UnitConverter/1 -> convert_in/1
  EM1ReqTorqLimBrk/1 -> UnitConverter/1

== system halin/HAL_IN/CAN1/EMC1_EM1/EM1ReqTorqLimDriv ==
  EM1ReqTorqLimDriv : Inport
  UnitConverter : DataTypeConversion  OutDataTypeStr=uint8
  convert_in : FVT_lib/hal/convert_in  gain=1  offset=-125
  VHAL_EM1ReqTorqLimDriv_pct : Outport
  wires:
  convert_in/1 -> VHAL_EM1ReqTorqLimDriv_pct/1
  UnitConverter/1 -> convert_in/1
  EM1ReqTorqLimDriv/1 -> UnitConverter/1

== system halin/HAL_IN/CAN1/HRW/WhlSpeedFL ==
  WhlSpeed_FL : Inport
  UnitConverter : DataTypeConversion  OutDataTypeStr=uint16
  convert_in : FVT_lib/hal/convert_in  gain=0.0039062  offset=0
  VHAL_WhlSpeedFL_kph : Outport
  wires:
  convert_in/1 -> VHAL_WhlSpeedFL_kph/1
  UnitConverter/1 -> convert_in/1
  WhlSpeed_FL/1 -> UnitConverter/1

== system halin/HAL_IN/CAN1/TC1/DrivDirF ==
  DrivDirF : Inport
  UnitConverter : DataTypeConversion  OutDataTypeStr=uint8
  VHAL_DrivDirF_enum : Outport
  wires:
  UnitConverter/1 -> VHAL_DrivDirF_enum/1
  DrivDirF/1 -> UnitConverter/1

== system halin/HAL_IN/CAN1/TC1/TransReqGear ==
  TransReqGear : Inport
  UnitConverter : DataTypeConversion  OutDataTypeStr=uint8
  VHAL_TransReqGear_enum : Outport
  wires:
  UnitConverter/1 -> VHAL_TransReqGear_enum/1
  TransReqGear/1 -> UnitConverter/1

== system halin/HAL_IN/CAN2/IVI_C100_0/IVIACFanSpdReqCmd ==
  IVI_ACFanSpdReq_Cmd : Inport
  UnitConverter : DataTypeConversion  OutDataTypeStr=uint8
  VHAL_IVIACFanSpdReqCmd_enum : Outport
  wires:
  UnitConverter/1 -> VHAL_IVIACFanSpdReqCmd_enum/1
  IVI_ACFanSpdReq_Cmd/1 -> UnitConverter/1

== system halin/HAL_IN/CAN3/B2TM_Info/B2THVRlySta ==
  B2THVRlySta : Inport
  UnitConverter : DataTypeConversion  OutDataTypeStr=uint8
  VHAL_B2THVRlySta_enum : Outport
  wires:
  UnitConverter/1 -> VHAL_B2THVRlySta_enum/1
  B2THVRlySta/1 -> UnitConverter/1

== system halin/HAL_IN/CAN3/B2V_BattInfo1/B2VBI1BattType ==
  B2VBI1BattType : Inport
  UnitConverter : DataTypeConversion  OutDataTypeStr=uint8
  VHAL_B2VBI1BattType_enum : Outport
  wires:
  UnitConverter/1 -> VHAL_B2VBI1BattType_enum/1
  B2VBI1BattType/1 -> UnitConverter/1

== system halin/HAL_IN/CAN3/B2V_CurrentLimit/B2VAPlsDischgCurr ==
  B2VAPlsDischgCurr : Inport
  UnitConverter : DataTypeConversion  OutDataTypeStr=uint16
  convert_in : FVT_lib/hal/convert_in  gain=0.1  offset=0
  VHAL_B2VAPlsDischgCurr_A : Outport
  wires:
  convert_in/1 -> VHAL_B2VAPlsDischgCurr_A/1
  UnitConverter/1 -> convert_in/1
  B2VAPlsDischgCurr/1 -> UnitConverter/1

== system halin/HAL_IN/CAN3/B2V_CurrentLimit/B2VAvaPlsChgCurr ==
  B2VAvaPlsChgCurr : Inport
  UnitConverter : DataTypeConversion  OutDataTypeStr=uint16
  convert_in : FVT_lib/hal/convert_in  gain=0.1  offset=0
  VHAL_B2VAvaPlsChgCurr_A : Outport
  wires:
  convert_in/1 -> VHAL_B2VAvaPlsChgCurr_A/1
  UnitConverter/1 -> convert_in/1
  B2VAvaPlsChgCurr/1 -> UnitConverter/1

== system halin/HAL_IN/CAN3/B2V_Fult1_32960/B2VHVILFault ==
  B2VHVILFault : Inport
  UnitConverter : DataTypeConversion  OutDataTypeStr=uint8
  VHAL_B2VHVILFault_flg : Outport
  wires:
  UnitConverter/1 -> VHAL_B2VHVILFault_flg/1
  B2VHVILFault/1 -> UnitConverter/1

== system halin/HAL_IN/CAN3/B2V_ST1/B2VACChgConnSta ==
  B2VACChgConnSta : Inport
  UnitConverter : DataTypeConversion  OutDataTypeStr=uint8
  VHAL_B2VACChgConnSta_flg : Outport
  wires:
  UnitConverter/1 -> VHAL_B2VACChgConnSta_flg/1
  B2VACChgConnSta/1 -> UnitConverter/1

== system halin/HAL_IN/CAN3/B2V_ST1/B2VACChgNegRlySta ==
  B2VACChgNegRlySta : Inport
  UnitConverter : DataTypeConversion  OutDataTypeStr=uint8
  VHAL_B2VACChgNegRlySta_enum : Outport
  wires:
  UnitConverter/1 -> VHAL_B2VACChgNegRlySta_enum/1
  B2VACChgNegRlySta/1 -> UnitConverter/1

== system halin/HAL_IN/CAN3/B2V_ST1/B2VACChgPosRlySta ==
  B2VACChgPosRlySta : Inport
  UnitConverter : DataTypeConversion  OutDataTypeStr=uint8
  VHAL_B2VACChgPosRlySta_enum : Outport
  wires:
  UnitConverter/1 -> VHAL_B2VACChgPosRlySta_enum/1
  B2VACChgPosRlySta/1 -> UnitConverter/1

== system halin/HAL_IN/CAN3/B2V_ST1/B2VBMUHVSta ==
  B2VBMUHVSta : Inport
  UnitConverter : DataTypeConversion  OutDataTypeStr=uint8
  VHAL_B2VBMUHVSta_enum : Outport
  wires:
  UnitConverter/1 -> VHAL_B2VBMUHVSta_enum/1
  B2VBMUHVSta/1 -> UnitConverter/1

== system halin/HAL_IN/CAN3/B2V_ST1/B2VChgMode ==
  B2VChgMode : Inport
  UnitConverter : DataTypeConversion  OutDataTypeStr=uint16
  VHAL_B2VChgMode_enum : Outport
  wires:
  UnitConverter/1 -> VHAL_B2VChgMode_enum/1
  B2VChgMode/1 -> UnitConverter/1

== system halin/HAL_IN/CAN3/B2V_ST1/B2VChgSta ==
  B2VChgSta : Inport
  UnitConverter : DataTypeConversion  OutDataTypeStr=uint8
  VHAL_B2VChgSta_enum : Outport
  wires:
  UnitConverter/1 -> VHAL_B2VChgSta_enum/1
  B2VChgSta/1 -> UnitConverter/1

== system halin/HAL_IN/CAN3/B2V_ST1/B2VDCChgConnSta ==
  B2VDCChgConnSta : Inport
  UnitConverter : DataTypeConversion  OutDataTypeStr=uint8
  VHAL_B2VDCChgConnSta_enum : Outport
  wires:
  UnitConverter/1 -> VHAL_B2VDCChgConnSta_enum/1
  B2VDCChgConnSta/1 -> UnitConverter/1

== system halin/HAL_IN/CAN3/B2V_ST1/B2VDCChgN1RlySta ==
  B2VDCChgN1RlySta : Inport
  UnitConverter : DataTypeConversion  OutDataTypeStr=uint8
  VHAL_B2VDCChgN1RlySta_enum : Outport
  wires:
  UnitConverter/1 -> VHAL_B2VDCChgN1RlySta_enum/1
  B2VDCChgN1RlySta/1 -> UnitConverter/1

== system halin/HAL_IN/CAN3/B2V_ST1/B2VDCChgP1RlySta ==
  B2VDCChgP1RlySta : Inport
  UnitConverter : DataTypeConversion  OutDataTypeStr=uint8
  VHAL_B2VDCChgP1RlySta_enum : Outport
  wires:
  UnitConverter/1 -> VHAL_B2VDCChgP1RlySta_enum/1
  B2VDCChgP1RlySta/1 -> UnitConverter/1

== system halin/HAL_IN/CAN3/B2V_ST1/B2VMainNegRlySta ==
  B2VMainNegRlySta : Inport
  UnitConverter : DataTypeConversion  OutDataTypeStr=uint8
  VHAL_B2VMainNegRlySta_enum : Outport
  wires:
  UnitConverter/1 -> VHAL_B2VMainNegRlySta_enum/1
  B2VMainNegRlySta/1 -> UnitConverter/1

== system halin/HAL_IN/CAN3/B2V_ST2/B2VFaultCode ==
  B2VFaultCode : Inport
  UnitConverter : DataTypeConversion  OutDataTypeStr=uint8
  VHAL_B2VFaultCode_enum : Outport
  wires:
  UnitConverter/1 -> VHAL_B2VFaultCode_enum/1
  B2VFaultCode/1 -> UnitConverter/1

== system halin/HAL_IN/CAN3/B2V_ST2/B2VFaultLv ==
  B2VFaultLv : Inport
  UnitConverter : DataTypeConversion  OutDataTypeStr=uint8
  VHAL_B2VFaultLv_enum : Outport
  wires:
  UnitConverter/1 -> VHAL_B2VFaultLv_enum/1
  B2VFaultLv/1 -> UnitConverter/1

== system halin/HAL_IN/CAN3/B2V_ST2/B2VPackCurr ==
  B2VPackCurr : Inport
  UnitConverter : DataTypeConversion  OutDataTypeStr=uint16
  convert_in : FVT_lib/hal/convert_in  gain=0.1  offset=-1000
  VHAL_B2VPackCurr_A : Outport
  wires:
  convert_in/1 -> VHAL_B2VPackCurr_A/1
  UnitConverter/1 -> convert_in/1
  B2VPackCurr/1 -> UnitConverter/1

== system halin/HAL_IN/CAN3/B2V_ST2/B2VPackInsideVol ==
  B2VPackInsideVol : Inport
  UnitConverter : DataTypeConversion  OutDataTypeStr=uint16
  convert_in : FVT_lib/hal/convert_in  gain=0.1  offset=0
  VHAL_B2VPackInsideVol_V : Outport
  wires:
  convert_in/1 -> VHAL_B2VPackInsideVol_V/1
  UnitConverter/1 -> convert_in/1
  B2VPackInsideVol/1 -> UnitConverter/1

== system halin/HAL_IN/CAN3/B2V_ST2/B2VRqHVPwrOff ==
  B2VRqHVPwrOff : Inport
  UnitConverter : DataTypeConversion  OutDataTypeStr=uint8
  VHAL_B2VRqHVPwrOff_enum : Outport
  wires:
  UnitConverter/1 -> VHAL_B2VRqHVPwrOff_enum/1
  B2VRqHVPwrOff/1 -> UnitConverter/1

== system halin/HAL_IN/CAN3/B2V_ST2/B2VSOC ==
  B2VSOC : Inport
  UnitConverter : DataTypeConversion  OutDataTypeStr=uint8
  convert_in : FVT_lib/hal/convert_in  gain=0.4  offset=0
  VHAL_B2VSOC_pct : Outport
  wires:
  convert_in/1 -> VHAL_B2VSOC_pct/1
  UnitConverter/1 -> convert_in/1
  B2VSOC/1 -> UnitConverter/1

== system halin/HAL_IN/CAN3/B2V_ST4/B2VMinTempPos ==
  B2VMinTempPos : Inport
  UnitConverter : DataTypeConversion  OutDataTypeStr=uint8
  VHAL_B2VMinTempPos_enum : Outport
  wires:
  UnitConverter/1 -> VHAL_B2VMinTempPos_enum/1
  B2VMinTempPos/1 -> UnitConverter/1

== system halin/HAL_IN/CAN3/B2V_ST5/B2VCellMinVol ==
  B2VCellMinVol : Inport
  UnitConverter : DataTypeConversion  OutDataTypeStr=uint16
  convert_in : FVT_lib/hal/convert_in  gain=0.001  offset=0
  VHAL_B2VCellMinVol_V : Outport
  wires:
  convert_in/1 -> VHAL_B2VCellMinVol_V/1
  UnitConverter/1 -> convert_in/1
  B2VCellMinVol/1 -> UnitConverter/1

== system halin/HAL_IN/CAN3/EWP1/EWPPEFault ==
  EWPPEFault : Inport
  UnitConverter : DataTypeConversion  OutDataTypeStr=uint8
  VHAL_EWPPEFault_enum : Outport
  wires:
  UnitConverter/1 -> VHAL_EWPPEFault_enum/1
  EWPPEFault/1 -> UnitConverter/1

== system halin/HAL_IN/CAN3/TM_MCUSta1/AtvDisChgEnFbk ==
  AtvDisChgEnFbk : Inport
  UnitConverter : DataTypeConversion  OutDataTypeStr=uint8
  VHAL_AtvDisChgEnFbk_flg : Outport
  wires:
  UnitConverter/1 -> VHAL_AtvDisChgEnFbk_flg/1
  AtvDisChgEnFbk/1 -> UnitConverter/1

== system halin/HAL_IN/CAN3/TM_MCUSta1/MCUCtrlMdSta ==
  MCUCtrlMdSta : Inport
  UnitConverter : DataTypeConversion  OutDataTypeStr=uint8
  VHAL_MCUCtrlMdSta_enum : Outport
  wires:
  UnitConverter/1 -> VHAL_MCUCtrlMdSta_enum/1
  MCUCtrlMdSta/1 -> UnitConverter/1

== system halin/HAL_IN/CAN3/TM_MCUSta1/MCUIGBTEnFbk ==
  MCUIGBTEnFbk : Inport
  UnitConverter : DataTypeConversion  OutDataTypeStr=uint8
  VHAL_MCUIGBTEnFbk_flg : Outport
  wires:
  UnitConverter/1 -> VHAL_MCUIGBTEnFbk_flg/1
  MCUIGBTEnFbk/1 -> UnitConverter/1

== system halin/HAL_IN/CAN3/TM_MCUSta1/MotorSpd ==
  MotorSpd : Inport
  UnitConverter : DataTypeConversion  OutDataTypeStr=uint16
  convert_in : FVT_lib/hal/convert_in  gain=1  offset=-15000
  VHAL_MotorSpd_rpm : Outport
  wires:
  convert_in/1 -> VHAL_MotorSpd_rpm/1
  UnitConverter/1 -> convert_in/1
  MotorSpd/1 -> UnitConverter/1

== system halin/HAL_IN/CAN3/TM_MCUSta1/MotorTrq ==
  MotorTrq : Inport
  UnitConverter : DataTypeConversion  OutDataTypeStr=uint16
  convert_in : FVT_lib/hal/convert_in  gain=1  offset=-5000
  VHAL_MotorTrq_Nm : Outport
  wires:
  convert_in/1 -> VHAL_MotorTrq_Nm/1
  UnitConverter/1 -> convert_in/1
  MotorTrq/1 -> UnitConverter/1

== system halin/HAL_IN/CAN3/TM_MCUSta2/MCUFailGrade ==
  MCUFailGrade : Inport
  UnitConverter : DataTypeConversion  OutDataTypeStr=uint8
  VHAL_MCUFailGrade_enum : Outport
  wires:
  UnitConverter/1 -> VHAL_MCUFailGrade_enum/1
  MCUFailGrade/1 -> UnitConverter/1

== system halin/HAL_IN/CAN3/TM_MCUSta2/MCUTemp ==
  MCUTemp : Inport
  UnitConverter : DataTypeConversion  OutDataTypeStr=uint8
  convert_in : FVT_lib/hal/convert_in  gain=1  offset=-40
  VHAL_MCUTemp_C : Outport
  wires:
  convert_in/1 -> VHAL_MCUTemp_C/1
  UnitConverter/1 -> convert_in/1
  MCUTemp/1 -> UnitConverter/1

== system halin/HAL_IN/CAN3/TM_MCUSta2/MCUTrqLimHi ==
  MCUTrqLimHi : Inport
  UnitConverter : DataTypeConversion  OutDataTypeStr=uint16
  VHAL_MCUTrqLimHi_Nm : Outport
  wires:
  UnitConverter/1 -> VHAL_MCUTrqLimHi_Nm/1
  MCUTrqLimHi/1 -> UnitConverter/1

== system halin/HAL_IN/CAN3/TM_MCUSta2/MCUTrqLimLo ==
  MCUTrqLimLo : Inport
  UnitConverter : DataTypeConversion  OutDataTypeStr=uint16
  convert_in : FVT_lib/hal/convert_in  gain=1  offset=-5000
  VHAL_MCUTrqLimLo_Nm : Outport
  wires:
  convert_in/1 -> VHAL_MCUTrqLimLo_Nm/1
  UnitConverter/1 -> convert_in/1
  MCUTrqLimLo/1 -> UnitConverter/1

== system halin/HAL_IN/CAN3/TM_MCUSta2/MotorTemp ==
  MotorTemp : Inport
  UnitConverter : DataTypeConversion  OutDataTypeStr=uint8
  convert_in : FVT_lib/hal/convert_in  gain=1  offset=-40
  VHAL_MotorTemp_C : Outport
  wires:
  convert_in/1 -> VHAL_MotorTemp_C/1
  UnitConverter/1 -> convert_in/1
  MotorTemp/1 -> UnitConverter/1

== system halin/HAL_IN/CAN3/TM_MCUSta3/MCUDCCur ==
  MCUDCCur : Inport
  UnitConverter : DataTypeConversion  OutDataTypeStr=uint16
  convert_in : FVT_lib/hal/convert_in  gain=1  offset=-1000
  VHAL_MCUDCCur_A : Outport
  wires:
  convert_in/1 -> VHAL_MCUDCCur_A/1
  UnitConverter/1 -> convert_in/1
  MCUDCCur/1 -> UnitConverter/1

== system halin/HAL_IN/CAN3/TM_MCUSta3/MCUDCVol ==
  MCUDCVol : Inport
  UnitConverter : DataTypeConversion  OutDataTypeStr=uint16
  convert_in : FVT_lib/hal/convert_in  gain=0.1  offset=0
  VHAL_MCUDCVol_V : Outport
  wires:
  convert_in/1 -> VHAL_MCUDCVol_V/1
  UnitConverter/1 -> convert_in/1
  MCUDCVol/1 -> UnitConverter/1

== system halin/HAL_IN/CAN3/TM_MCUSta3/MCUFailCode ==
  MCUFailCode : Inport
  UnitConverter : DataTypeConversion  OutDataTypeStr=uint8
  VHAL_MCUFailCode_enum : Outport
  wires:
  UnitConverter/1 -> VHAL_MCUFailCode_enum/1
  MCUFailCode/1 -> UnitConverter/1

== system halin/HAL_IN/CAN4/ZFR_C100_0/ParkBrakeSW ==
  ParkBrakeSW : Inport
  UnitConverter : DataTypeConversion  OutDataTypeStr=uint8
  VHAL_ParkBrakeSW_enum : Outport
  wires:
  UnitConverter/1 -> VHAL_ParkBrakeSW_enum/1
  ParkBrakeSW/1 -> UnitConverter/1

== system halin/HAL_IN/CAN4/ZFR_CE100_0/AirPressureFC2 ==
  AirPressureFC2 : Inport
  UnitConverter : DataTypeConversion  OutDataTypeStr=uint8
  convert_in : FVT_lib/hal/convert_in  gain=8  offset=0
  VHAL_AirPressureFC2_kPa : Outport
  wires:
  convert_in/1 -> VHAL_AirPressureFC2_kPa/1
  UnitConverter/1 -> convert_in/1
  AirPressureFC2/1 -> UnitConverter/1

== system halin/HAL_IN/CAN4/ZFR_CE100_0/ZFRBCMAutoLightSWSta ==
  ZFR_BCM_AutoLightSW_Sta : Inport
  UnitConverter : DataTypeConversion  OutDataTypeStr=uint8
  VHAL_ZFRBCMAutoLightSWSta_flg : Outport
  wires:
  UnitConverter/1 -> VHAL_ZFRBCMAutoLightSWSta_flg/1
  ZFR_BCM_AutoLightSW_Sta/1 -> UnitConverter/1

== system halin/HAL_IN/CAN4/ZFR_CE100_0/ZFRBCMBrakeSta ==
  ZFR_BCM_Brake_Sta : Inport
  UnitConverter : DataTypeConversion  OutDataTypeStr=uint8
  VHAL_ZFRBCMBrakeSta_flg : Outport
  wires:
  UnitConverter/1 -> VHAL_ZFRBCMBrakeSta_flg/1
  ZFR_BCM_Brake_Sta/1 -> UnitConverter/1

== system halin/HAL_IN/CAN4/ZFR_CE100_0/ZFRBCMHBeamSWSta ==
  ZFR_BCM_HBeamSW_Sta : Inport
  UnitConverter : DataTypeConversion  OutDataTypeStr=uint8
  VHAL_ZFRBCMHBeamSWSta_flg : Outport
  wires:
  UnitConverter/1 -> VHAL_ZFRBCMHBeamSWSta_flg/1
  ZFR_BCM_HBeamSW_Sta/1 -> UnitConverter/1

== system halin/HAL_IN/CAN4/ZFR_CE100_0/ZFRBCMHeadLpSWSta ==
  ZFR_BCM_HeadLpSW_Sta : Inport
  UnitConverter : DataTypeConversion  OutDataTypeStr=uint8
  VHAL_ZFRBCMHeadLpSWSta_flg : Outport
  wires:
  UnitConverter/1 -> VHAL_ZFRBCMHeadLpSWSta_flg/1
  ZFR_BCM_HeadLpSW_Sta/1 -> UnitConverter/1

== system halin/HAL_IN/CAN4/ZFR_CE100_0/ZFRBCMLFTurnLpCSta ==
  ZFR_BCM_LFTurnLpC_Sta : Inport
  UnitConverter : DataTypeConversion  OutDataTypeStr=uint8
  convert_in : FVT_lib/hal/convert_in  gain=0.025  offset=0
  VHAL_ZFRBCMLFTurnLpCSta_A : Outport
  wires:
  convert_in/1 -> VHAL_ZFRBCMLFTurnLpCSta_A/1
  UnitConverter/1 -> convert_in/1
  ZFR_BCM_LFTurnLpC_Sta/1 -> UnitConverter/1

== system halin/HAL_IN/CAN4/ZFR_CE100_0/ZFRBCMLightSensorVSta ==
  ZFR_BCM_LightSensorV_Sta : Inport
  UnitConverter : DataTypeConversion  OutDataTypeStr=uint8
  convert_in : FVT_lib/hal/convert_in  gain=0.0196  offset=0
  VHAL_ZFRBCMLightSensorVSta_V : Outport
  wires:
  convert_in/1 -> VHAL_ZFRBCMLightSensorVSta_V/1
  UnitConverter/1 -> convert_in/1
  ZFR_BCM_LightSensorV_Sta/1 -> UnitConverter/1

== system halin/HAL_IN/CAN4/ZFR_CE100_0/ZFRBCMPLampSta ==
  ZFR_BCM_PLamp_Sta : Inport
  UnitConverter : DataTypeConversion  OutDataTypeStr=uint8
  VHAL_ZFRBCMPLampSta_flg : Outport
  wires:
  UnitConverter/1 -> VHAL_ZFRBCMPLampSta_flg/1
  ZFR_BCM_PLamp_Sta/1 -> UnitConverter/1

== system halin/HAL_IN/CAN4/ZFR_CE100_0/ZFRBCMRFTurnLpCSta ==
  ZFR_BCM_RFTurnLpC_Sta : Inport
  UnitConverter : DataTypeConversion  OutDataTypeStr=uint8
  convert_in : FVT_lib/hal/convert_in  gain=0.025  offset=0
  VHAL_ZFRBCMRFTurnLpCSta_A : Outport
  wires:
  convert_in/1 -> VHAL_ZFRBCMRFTurnLpCSta_A/1
  UnitConverter/1 -> convert_in/1
  ZFR_BCM_RFTurnLpC_Sta/1 -> UnitConverter/1

== system halin/HAL_IN/CAN4/ZFR_CE100_0/ZFRBCMRFogLpSWSta ==
  ZFR_BCM_RFogLp_SW_Sta : Inport
  UnitConverter : DataTypeConversion  OutDataTypeStr=uint8
  VHAL_ZFRBCMRFogLpSWSta_flg : Outport
  wires:
  UnitConverter/1 -> VHAL_ZFRBCMRFogLpSWSta_flg/1
  ZFR_BCM_RFogLp_SW_Sta/1 -> UnitConverter/1

== system halin/HAL_IN/CAN4/ZFR_CE100_0/ZFRBCMSeatbeltSta ==
  ZFR_BCM_Seatbelt_Sta : Inport
  UnitConverter : DataTypeConversion  OutDataTypeStr=uint8
  VHAL_ZFRBCMSeatbeltSta_flg : Outport
  wires:
  UnitConverter/1 -> VHAL_ZFRBCMSeatbeltSta_flg/1
  ZFR_BCM_Seatbelt_Sta/1 -> UnitConverter/1

== system halin/HAL_IN/CAN4/ZFR_CE100_0/ZFRBCMWasherSWSta ==
  ZFR_BCM_WasherSW_Sta : Inport
  UnitConverter : DataTypeConversion  OutDataTypeStr=uint8
  VHAL_ZFRBCMWasherSWSta_flg : Outport
  wires:
  UnitConverter/1 -> VHAL_ZFRBCMWasherSWSta_flg/1
  ZFR_BCM_WasherSW_Sta/1 -> UnitConverter/1

== system halin/HAL_IN/CAN4/ZFR_CE100_0/ZFRBCMWiperASSta ==
  ZFR_BCM_WiperAS_Sta : Inport
  UnitConverter : DataTypeConversion  OutDataTypeStr=uint8
  VHAL_ZFRBCMWiperASSta_flg : Outport
  wires:
  UnitConverter/1 -> VHAL_ZFRBCMWiperASSta_flg/1
  ZFR_BCM_WiperAS_Sta/1 -> UnitConverter/1

== system halin/HAL_IN/CAN4/ZFR_CE100_0/ZFRBCMWiperHSWSta ==
  ZFR_BCM_WiperHSW_Sta : Inport
  UnitConverter : DataTypeConversion  OutDataTypeStr=uint8
  VHAL_ZFRBCMWiperHSWSta_flg : Outport
  wires:
  UnitConverter/1 -> VHAL_ZFRBCMWiperHSWSta_flg/1
  ZFR_BCM_WiperHSW_Sta/1 -> UnitConverter/1

== system halin/HAL_IN/CAN4/ZFR_CE100_0/ZFRBCMWiperLSWSta ==
  ZFR_BCM_WiperLSW_Sta : Inport
  UnitConverter : DataTypeConversion  OutDataTypeStr=uint8
  VHAL_ZFRBCMWiperLSWSta_flg : Outport
  wires:
  UnitConverter/1 -> VHAL_ZFRBCMWiperLSWSta_flg/1
  ZFR_BCM_WiperLSW_Sta/1 -> UnitConverter/1

== system halin/HAL_IN/CAN4/ZRR_CE100_0/ZRRBCMAllDoorSta ==
  ZRR_BCM_AllDoor_Sta : Inport
  UnitConverter : DataTypeConversion  OutDataTypeStr=uint8
  VHAL_ZRRBCMAllDoorSta_enum : Outport
  wires:
  UnitConverter/1 -> VHAL_ZRRBCMAllDoorSta_enum/1
  ZRR_BCM_AllDoor_Sta/1 -> UnitConverter/1

== system halin/HAL_IN/CAN4/ZRR_CE100_1/AirPressurePC3 ==
  AirPressurePC3 : Inport
  UnitConverter : DataTypeConversion  OutDataTypeStr=uint8
  convert_in : FVT_lib/hal/convert_in  gain=8  offset=0
  VHAL_AirPressurePC3_kPa : Outport
  wires:
  convert_in/1 -> VHAL_AirPressurePC3_kPa/1
  UnitConverter/1 -> convert_in/1
  AirPressurePC3/1 -> UnitConverter/1

== system halin/HAL_IN/CAN4/ZRR_CE100_1/AirPressureRC1 ==
  AirPressureRC1 : Inport
  UnitConverter : DataTypeConversion  OutDataTypeStr=uint8
  convert_in : FVT_lib/hal/convert_in  gain=8  offset=0
  VHAL_AirPressureRC1_kPa : Outport
  wires:
  convert_in/1 -> VHAL_AirPressureRC1_kPa/1
  UnitConverter/1 -> convert_in/1
  AirPressureRC1/1 -> UnitConverter/1

== system halin/HAL_IN/CAN4/ZRR_CE100_1/FDCCHASSISVCUEACPressSta ==
  FDC_CHASSIS_VCUEACPress_Sta : Inport
  UnitConverter : DataTypeConversion  OutDataTypeStr=uint8
  VHAL_FDCCHASSISVCUEACPressSta_flg : Outport
  wires:
  UnitConverter/1 -> VHAL_FDCCHASSISVCUEACPressSta_flg/1
  FDC_CHASSIS_VCUEACPress_Sta/1 -> UnitConverter/1

== system halin/HAL_IN/CAN4/ZRR_CE100_1/ZRRBCMCallingSWSta ==
  ZRR_BCM_CallingSW_Sta : Inport
  UnitConverter : DataTypeConversion  OutDataTypeStr=uint8
  VHAL_ZRRBCMCallingSWSta_flg : Outport
  wires:
  UnitConverter/1 -> VHAL_ZRRBCMCallingSWSta_flg/1
  ZRR_BCM_CallingSW_Sta/1 -> UnitConverter/1

== system halin/HAL_IN/CAN4/ZRR_CE100_1/ZRRBCMLRTurnLpCSta ==
  ZRR_BCM_LRTurnLpC_Sta : Inport
  UnitConverter : DataTypeConversion  OutDataTypeStr=uint8
  convert_in : FVT_lib/hal/convert_in  gain=0.025  offset=0
  VHAL_ZRRBCMLRTurnLpCSta_A : Outport
  wires:
  convert_in/1 -> VHAL_ZRRBCMLRTurnLpCSta_A/1
  UnitConverter/1 -> convert_in/1
  ZRR_BCM_LRTurnLpC_Sta/1 -> UnitConverter/1
